simulink model "task1"  (R2024a)
settings: Solver=ode45  StartTime=0.0  StopTime=8  MaxStep=1e-3  RelTol=1e-3
values from neighbouring files (symbols this model uses):
  den_diff = [0.005 1]    [exp2_task1.m]    (also in task1_run.m)
  den_vartheta = [Td^2, 2*xid*Td, 1, 0]    [exp2_task1.m]    (also in task1_run.m)
  K_om = 0.20    (= 0.2)    [exp2_task1.m]    (also in task1_run.m)
  K_th = 3.0    (= 3)    [exp2_task1.m]    (also in task1_run.m)
  num_diff = [1 0]    [exp2_task1.m]    (also in task1_run.m)
  num_vartheta = [Kd*T1d, Kd]    [exp2_task1.m]    (also in task1_run.m)
  vartheta_cmd = deg2rad(5)    [exp2_task1.m]    (also in task1_run.m)
settings Model: Creator=taole  LastModifiedBy=taole

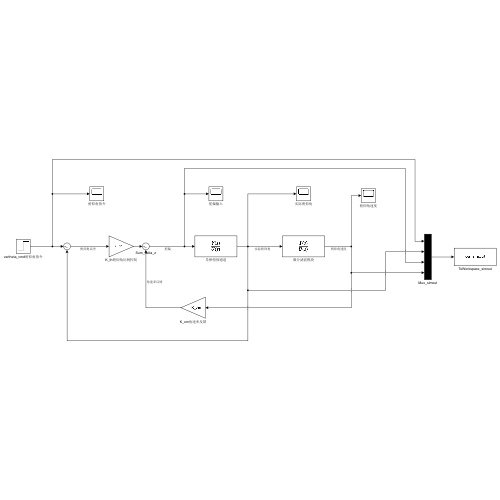
[thumbnail: Simulink's stored preview of the top-level diagram]
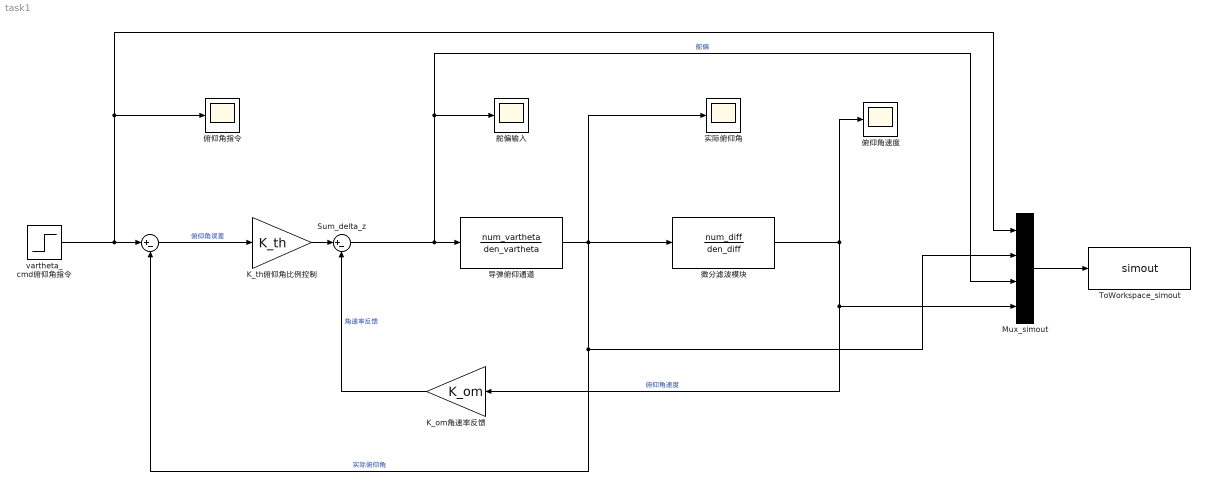
== system task1 ==
  " " : Sum  Inputs=|+-
  K_om角速率反馈 : Gain  Gain=K_om
  K_th俯仰角比例控制 : Gain  Gain=K_th
  Mux_simout : Mux
  Sum_delta_z : Sum  Inputs=|+-
  ToWorkspace_simout : ToWorkspace  VariableName=simout  SampleTime=-1
  vartheta_cmd俯仰角指令 : Step  Time=0  After=vartheta_cmd  SampleTime=0
  俯仰角指令 : Scope
  俯仰角速度 : Scope
  实际俯仰角 : Scope
  导弹俯仰通道 : TransferFcn  Numerator=num_vartheta  Denominator=den_vartheta
  微分滤波模块 : TransferFcn  Numerator=num_diff  Denominator=den_diff
  舵偏输入 : Scope
  wires:
  vartheta_cmd俯仰角指令/1 -> " "/1, 俯仰角指令/1, Mux_simout/1
  " "/1 -> K_th俯仰角比例控制/1  "俯仰角误差"
  K_th俯仰角比例控制/1 -> Sum_delta_z/1
  Sum_delta_z/1 -> 导弹俯仰通道/1, 舵偏输入/1, Mux_simout/3  "舵偏"
  导弹俯仰通道/1 -> " "/2, Mux_simout/2, 微分滤波模块/1, 实际俯仰角/1  "实际俯仰角"
  微分滤波模块/1 -> 俯仰角速度/1, K_om角速率反馈/1, Mux_simout/4  "俯仰角速度"
  K_om角速率反馈/1 -> Sum_delta_z/2  "角速率反馈"
  Mux_simout/1 -> ToWorkspace_simout/1
